simulink model "lab2_part1"  (R2025b)
settings: Solver=VariableStepAuto  StartTime=0.0  StopTime=30.0  RelTol=1e-10  AbsTol=1e-10
values from neighbouring files (symbols this model uses):
  A = [0 1; 0 -alpha_2/M]    [lab2.m]
  B = [0; alpha_1/M]    [lab2.m]
  K = [K1 K2]    [lab2.m]
settings Model: Creator=richardwu
settings RTWCC: GPUComputeCapability=3.5

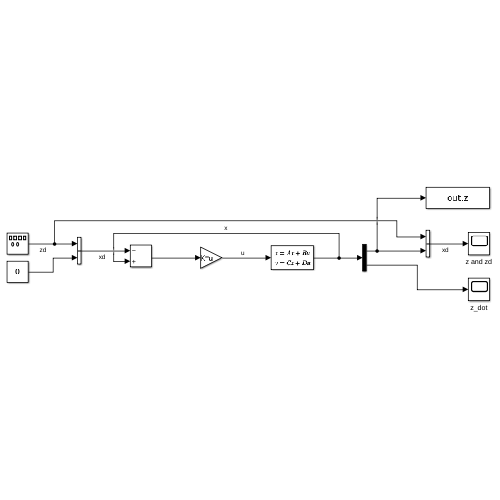
[thumbnail: Simulink's stored preview of the top-level diagram]
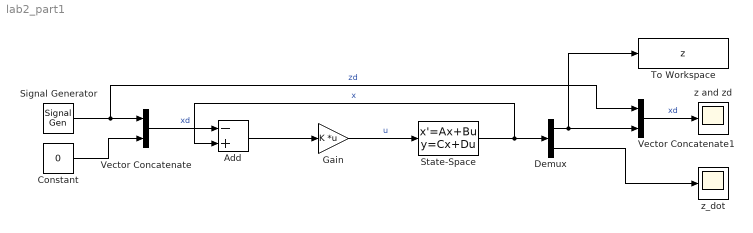
== system lab2_part1 ==
  Add : Sum  Inputs=-+
  Constant : Constant  Value=0
  Demux : Demux  Outputs=2
  Gain : Gain  Gain=K  Multiplication=Matrix(K*u)
  Signal Generator : SignalGenerator  WaveForm=square  Amplitude=0.03  Frequency=0.1
  State-Space : StateSpace  A=A  B=B  C=eye(2)  D=zeros(2,1)  InitialCondition=0
  To Workspace : ToWorkspace  VariableName=z  SaveFormat=Timeseries  SampleTime=-1
  Vector Concatenate : Concatenate
  Vector Concatenate1 : Concatenate
  z and zd : Scope
      settings: ActiveDisplayYMinimum=-0.68339904970330534  ActiveDisplayYMaximum=1.0690622136558607
  z_dot : Scope
      settings: ActiveDisplayYMinimum=-0.1491210480207934  ActiveDisplayYMaximum=0.17097659859496253
  wires:
  Signal Generator/1 -> Vector Concatenate1/1, Vector Concatenate/1  "zd"
  Constant/1 -> Vector Concatenate/2
  Vector Concatenate/1 -> Add/1  "xd"
  Add/1 -> Gain/1
  Gain/1 -> State-Space/1  "u"
  Vector Concatenate1/1 -> z and zd/1  "xd"
  Demux/1 -> To Workspace/1, Vector Concatenate1/2
  Demux/2 -> z_dot/1
  State-Space/1 -> Add/2, Demux/1  "x"
